simulink model "Kugle_sys8_block"  (R2018b)
settings: Solver=VariableStepAuto  StartTime=0.0  StopTime=10.0  RelTol=1e-3
settings Model: Creator=martinandersen  LastModifiedBy=martinandersen

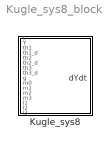
== system Kugle_sys8_block ==
  Kugle_sys8 : MATLAB Function  TreatAsAtomicUnit=on

== matlab function Kugle_sys8_block/Kugle_sys8 ==
  data: t input; dYdt output; Y input; th1 input; th1_d input; th2 input; th2_d input; th3 input; th3_d input; g input; m0 input; m1 input; m2 input; m3 input; l1 input; l2 input; l3 input
function dYdt = Kugle_sys8(t,Y,th1,th1_d,th2,th2_d,th3,th3_d,g,m0,m1,m2,m3,l1,l2,l3)
%#codegen

%    This function was generated by the Symbolic Math Toolbox version 8.2.
%    14-May-2019 11:55:54

dYdt = [Y(2);0.0];
